simulink model "Simulation_6DOFTesting02"  (R2024a)
settings: Solver=ode4  StartTime=initial_time  StopTime=final_time  FixedStep=timestep  RelTol=1e-3
values from neighbouring files (symbols this model uses):
  aEarth = 0    [CodeTesting_6DOF.m]    (also in Constants_6DOF.m = 6378137; Constants_6DOFTesting.m = 6378137)
  alphaArray = [-30, -25, -20, -15, -10, -5, 0, 5, 10, 15, 20, 25, 30]    [CodeTesting_6DOF.m]    (also in Constants_6DOF.m; Constants_6DOFTesting.m)
  altitudeArray = [0, 1000, 2000, 3000, 4000, 5000, 6000, 7000, 8000, 9000, 10000, 15000, 20000,      25000, 30000, 35000, 40000, 45000, 50000, 55000, 60000]    [CodeTesting_6DOF.m]    (also in Constants_6DOF.m; Constants_6DOFTesting.m)
  bEarth = 0    [CodeTesting_6DOF.m]    (also in Constants_6DOF.m = 6356752.3; Constants_6DOFTesting.m = 6356752.3)
  cD_3DArray = zeros(numAoAs, numMachs, numAltitudes)    [CodeTesting_6DOF.m]    (also in Constants_6DOF.m; Constants_6DOFTesting.m)
  cL_3DArray = zeros(numAoAs, numMachs, numAltitudes)    [CodeTesting_6DOF.m]    (also in Constants_6DOF.m; Constants_6DOFTesting.m)
  densityList = rhoList    [CodeTesting_6DOF.m]    (also in Constants_6DOF.m = usAtmosphere.x_; Constants_6DOFTesting.m = usAtmosphere.x_)
  height0 = 0    [Constants_6DOF.m]    (also in Constants_6DOFTesting.m = 5000)
  heightsList = usAtmosphere.Z    [CodeTesting_6DOF.m]    (also in Constants_6DOF.m; Constants_6DOFTesting.m)
  inertialPitch0 = deg2rad(inertialPitch0)    [Constants_6DOFTesting.m]
  inertialRoll0 = deg2rad(inertialRoll0)    [Constants_6DOFTesting.m]
  inertialYaw0 = deg2rad(inertialYaw0)    [Constants_6DOFTesting.m]
  initQuatVector0 = [e0; e1; e2; e3]    [Constants_6DOFTesting.m]
  Ixx = 10    [CodeTesting_6DOF.m]    (also in Constants_6DOF.m; Constants_6DOFTesting.m = 4.88094462)
  Ixz = 10    [CodeTesting_6DOF.m]    (also in Constants_6DOF.m = 1; Constants_6DOFTesting.m = 4.88094462)
  Iyy = 10    [CodeTesting_6DOF.m]    (also in Constants_6DOF.m; Constants_6DOFTesting.m = 4.88094462)
  Izz = 10    [CodeTesting_6DOF.m]    (also in Constants_6DOF.m; Constants_6DOFTesting.m = 4.88094462)
  latitude0 = pi/4    (= 0.785398163397)    [CodeTesting_6DOF.m]    (also in Constants_6DOF.m = deg2rad(latitude0); Constants_6DOFTesting.m = deg2rad(latitude0))
  longitude0 = pi/4    (= 0.785398163397)    [CodeTesting_6DOF.m]    (also in Constants_6DOF.m = deg2rad(longitude0); Constants_6DOFTesting.m = deg2rad(longitude0))
  m0 = 10    [CodeTesting_6DOF.m]    (also in Constants_6DOF.m = 50; Constants_6DOFTesting.m = 14.5939029)
  machArray = [0.5, 1.0, 1.5, 2.0, 2.5, 3.0, 3.5, 4.0, 4.5, 5.0, 5.5, 6.0, 6.5, 7.0, 7.5, 8.0,      8.5, 9.0, 9.5, 10.0]    [CodeTesting_6DOF.m]    (also in Constants_6DOF.m; Constants_6DOFTesting.m)
  omegaEarth = omega_earth    (= 7.2921159e-05)    [CodeTesting_6DOF.m]    (also in Constants_6DOF.m; Constants_6DOFTesting.m)
  p0Body = deg2rad(p0Body)    [Constants_6DOFTesting.m]
  pitchCharacteristicLength = 0.0    (= 0)    [Constants_6DOFTesting.m]
  q0Body = deg2rad(q0Body)    [Constants_6DOFTesting.m]
  r0Body = deg2rad(r0Body)    [Constants_6DOFTesting.m]
  rEarth = r_earth    (= 6371008.8)    [CodeTesting_6DOF.m]    (also in Constants_6DOF.m; Constants_6DOFTesting.m)
  rollCharacteristicLength = 0.0    (= 0)    [Constants_6DOFTesting.m]
  temperatureList = usAtmosphere.T    [CodeTesting_6DOF.m]    (also in Constants_6DOF.m; Constants_6DOFTesting.m)
  u0Body = 304.8    [Constants_6DOFTesting.m]
  v0Body = 0    [Constants_6DOFTesting.m]
  w0Body = -1 * w0Body    (= 0)    [Constants_6DOFTesting.m]
  wingArea = 0    [CodeTesting_6DOF.m]    (also in Constants_6DOF.m = 50; Constants_6DOFTesting.m = 0.09290304)
  yawCharacteristicLength = 0.0    (= 0)    [Constants_6DOFTesting.m]
undefined symbols (not defined in the file or in its folder): inertialX0, inertialY0, inertialZ0
libraries: simulink_extras x24
(part 2 of 2)

== matlab function Simulation_6DOFTesting02/Equations of Motion/Subsystem1/MATLAB Function1 ==
  data: angularRatesBody input; y output; quatRotBTN input
function y= fcn(angularRatesBody, quatRotBTN)

rotationMatrixIB = quatRotBTN;

angularRatesInertial =  angularRatesBody;

y = angularRatesInertial;

== matlab function Simulation_6DOFTesting02/Atmospheric Conditions/Mach ==
  data: v input; y output; r input; hList input; tempList input
function y = fcn(v, r, hList, tempList)

gamma = 1.4;
rGas = 287.05;

r = r / 10^3;

if r >= 0
    temp = interp1(hList, tempList, r);
    a = sqrt(gamma * rGas * temp);
    y = v/a;
else
    temp = 0;
    y = 0;
end

== matlab function Simulation_6DOFTesting02/Forces, Moments & their Coefficients/rollMoment ==
  data: rho input; y output; v input; A input; length input; rollCoeff input
function y = fcn(rho, v, A, length, rollCoeff)

rollMoment = 0.5 * rho * v^2 * A * rollCoeff * length;

y = rollMoment;

== matlab function Simulation_6DOFTesting02/Forces, Moments & their Coefficients/pitchMoment ==
  data: rho input; y output; v input; A input; length input; pitchCoeff input
function y = fcn(rho, v, A, length, pitchCoeff)

pitchMoment = 0.5 * rho * v^2 * A * length * pitchCoeff;

y = pitchMoment;

== matlab function Simulation_6DOFTesting02/Equations of Motion/Subsystem2/MATLAB Function ==
  data: quatVector input; y output
function y = fcn(quatVector)

lambda = 1000;

quatVectorNormalized = quatVector - lambda * (1 - norm(quatVector)^2 )^2;

normQuatVecCheck = norm(quatVectorNormalized);

y = quatVectorNormalized;

== matlab function Simulation_6DOFTesting02/Forces, Moments & their Coefficients/yawMoment ==
  data: rho input; y output; v input; A input; length input; yawCoeff input
function y = fcn(rho, v, A, length, yawCoeff)

yawMoment = 0.5 * rho * v^2 * A * length * yawCoeff;

y = yawMoment;

== matlab function Simulation_6DOFTesting02/Equations of Motion/Subsystem/Subsystem4/uDot_Body ==
  data: Fx input; y output; m input; r input; v input; q input; w input
function y = fcn(Fx, m, r, v, q, w)

uDot_Wind = (Fx/m) + r * v - q * w;

y = uDot_Wind;

== matlab function Simulation_6DOFTesting02/Equations of Motion/Subsystem/Subsystem3/vDot_Body ==
  data: Fy input; y output; m input; p input; w input; r input; u input
function y = fcn(Fy, m, p, w, r,  u)

vDot_Wind = (Fy / m) + p * w - r * u;

y = vDot_Wind;

== matlab function Simulation_6DOFTesting02/Equations of Motion/Subsystem/Subsystem2/wDot_Body ==
  data: Fz input; y output; m input; q input; u input; p input; v input
function y = fcn(Fz, m, q, u, p, v)

vDot_Wind = (Fz / m) + q * u - p * v;

y = vDot_Wind;

== matlab function Simulation_6DOFTesting02/Equations of Motion/Subsystem/Subsystem/pDot_Body ==
  data: rollMoment input; y output; Ixx input; Ixz input; rDot_Body input; Izz input; Iyy input; q input; r input; p input
function y = fcn(rollMoment, Ixx, Ixz, rDot_Body, Izz, Iyy, q, r, p)

pDot_Wind = (1/Ixx) * (Ixz * rDot_Body - (Izz - Iyy) * q * r + Ixz * p * q - rollMoment);

y = pDot_Wind;

== matlab function Simulation_6DOFTesting02/Forces, Moments & their Coefficients/Subsystem1/MATLAB Function ==
  data: m input; y output; g input; quatRotBTN input
function y = fcn(m, g, quatRotBTN)

inertialGravity = [0; 0; m * g];

rotationMatrixBI = quatRotBTN;

rotationBI = inv(rotationMatrixBI);

bodyGravity = rotationBI * inertialGravity;

y = bodyGravity;

== matlab function Simulation_6DOFTesting02/Equations of Motion/Subsystem/qBody/qDot_Body ==
  data: pitchMoment input; Iyy input; Izz input; y output; Ixx input; p input; r input; Ixz input
function y = fcn(pitchMoment, Iyy, Izz, Ixx, p, r, Ixz)

qDot_Wind = (1/Iyy) * ( -pitchMoment - (Ixx - Izz) * p * r - Ixz * (p^2 - r^2));

y = qDot_Wind;

== matlab function Simulation_6DOFTesting02/Equations of Motion/Subsystem/rBody/rDot_Body ==
  data: yawMoment input; Izz input; Ixz input; pDot_Body input; y output; Ixx input; Iyy input; p input; q input; r input
function y = fcn(yawMoment, Izz, Ixz, pDot_Body, Ixx, Iyy, p, q, r)

rDot_Wind = (1/Izz) * (Ixz * pDot_Body - (Iyy - Ixx) * p * q - Ixz * q * r - yawMoment);

y = rDot_Wind;

== matlab function Simulation_6DOFTesting02/Atmospheric Conditions/g ==
  data: y output; r input
function y = fcn(r)

mu_earth = 3.986004418 * 10^14;
rE = 6378140;

y = mu_earth / (rE + r)^2;

== matlab function Simulation_6DOFTesting02/Atmospheric Conditions/rho ==
  data: rhoList input; hList input; r input; y output
function y = fcn(rhoList, hList, r)

r = r / 10^3;

if r >= 0
    density = interp1(hList, rhoList, r);
else
    density = 0;
end


y = density;

== matlab function Simulation_6DOFTesting02/Coordinate Transformations/Subsystem/velocity ==
  data: u input; y output; v input; w input
function y = fcn(u, v, w)

velocity = sqrt(u^2 + v^2 + w^2);

y = velocity;

== matlab function Simulation_6DOFTesting02/Constants & Aircraft Parameters/mass ==
  data: t input; y output; thrustBurnRate input; m0 input
function y = fcn(t, thrustBurnRate, m0)

mass = m0 - thrustBurnRate * t;

y = mass;

== matlab function Simulation_6DOFTesting02/Forces, Moments & their Coefficients/Subsystem/AoA1 ==
  data: u input; y output; v input; w input
function y = fcn(u, v, w)

%AoA = -1 * asin(w / sqrt(u^2 + v^2 + w^2) );
AoA = atan(-w / u);

y = AoA;

== matlab function Simulation_6DOFTesting02/Control Surfaces/bankAngle ==
  data: t input; y output
function y = fcn(t)

bankAngle = 0;

y = bankAngle;

== matlab function Simulation_6DOFTesting02/Control Surfaces/flightPathAngle ==
  data: t input; y output
function y = fcn(t)

flightPathAngle = 0;

y = flightPathAngle;

== matlab function Simulation_6DOFTesting02/Control Surfaces/pitchSurfaceDeflection ==
  data: t input; y output
function y = fcn(t)

pitchSurfaceDeflection = 0.0;

if t > 5 && t < 15
    pitchSurfaceDeflection = 0.001;
end

if t > 20 && t < 25
    pitchSurfaceDeflection = -0.001;
end


y = pitchSurfaceDeflection;

== matlab function Simulation_6DOFTesting02/Equations of Motion/Subsystem2/quatVectorDot ==
  data: quatVector input; y output; p input; q input; r input
function y = fcn(quatVector, p, q, r)



row1 = 1/2 * [0 -p -q -r];
row2 = 1/2 * [p 0 r -q];
row3 = 1/2 * [q -r 0 p];
row4 = 1/2 * [r q -p 0];


updateMatrix = [row1; row2; row3; row4];

quatDotVector = (updateMatrix * quatVector); 
%Normalize post integrtation - lambda * (1 - norm(quatVector)^2 )^2;

y = quatDotVector;

== matlab function Simulation_6DOFTesting02/Forces, Moments & their Coefficients/rollCoeff ==
  data: rollSurfaceDeflection input; y output
function y = fcn(rollSurfaceDeflection)

staticRollCoeff = rollSurfaceDeflection;
dynamicRollCoeff = 0.0;

rollCoeff = staticRollCoeff + dynamicRollCoeff;

y = rollCoeff;

== matlab function Simulation_6DOFTesting02/Forces, Moments & their Coefficients/pitchCoeff ==
  data: pitchSurfaceDeflection input; y output
function y = fcn(pitchSurfaceDeflection)

staticPitchCoeff = pitchSurfaceDeflection;
dynamicPitchCoeff = 0.0;

pitchCoeff = staticPitchCoeff + dynamicPitchCoeff;

y = pitchCoeff;

== matlab function Simulation_6DOFTesting02/Forces, Moments & their Coefficients/yawCoeff ==
  data: yawSurfaceDeflection input; y output
function y = fcn(yawSurfaceDeflection)

staticYawCoeff = yawSurfaceDeflection;
dynamicYawCoeff = 0.0;

yawCoeff = staticYawCoeff + dynamicYawCoeff;

y = yawCoeff;

== matlab function Simulation_6DOFTesting02/Constants & Aircraft Parameters/thrustBurnRate ==
  data: t input; y output
function y = fcn(t)

thrustBurnRate = 0;

y = thrustBurnRate;

== matlab function Simulation_6DOFTesting02/Forces, Moments & their Coefficients/Fx ==
  data: thrustX input; y output; gravityX input; dragX input
function y = fcn(thrustX, gravityX, dragX)

xForce = thrustX - gravityX - dragX;

y = xForce;

== matlab function Simulation_6DOFTesting02/Forces, Moments & their Coefficients/Fy ==
  data: thrustY input; y output; gravityY input
function y = fcn(thrustY, gravityY)

yForce = thrustY - gravityY;

y = yForce;

== matlab function Simulation_6DOFTesting02/Forces, Moments & their Coefficients/Fz ==
  data: thrustZ input; y output; gravityZ input; liftZ input
function y = fcn(thrustZ, gravityZ, liftZ)

zForce = thrustZ + gravityZ - liftZ;

y = zForce;

== matlab function Simulation_6DOFTesting02/Forces, Moments & their Coefficients/MATLAB Function ==
  data: thrustX input; y output; thrustY input; thrustZ input
function y = fcn(thrustX, thrustY, thrustZ)

thrustMagnitude = sqrt(thrustX^2 + thrustY^2 + thrustZ^2);

y = thrustMagnitude;

== matlab function Simulation_6DOFTesting02/Forces, Moments & their Coefficients/MATLAB Function1 ==
  data: forceVector input; y output; quatRotWTB input
function y = fcn(forceVector, quatRotWTB)

rotationMatrix = quatRotWTB;

rotatedForceVector = rotationMatrix * forceVector;

y = rotatedForceVector;

== matlab function Simulation_6DOFTesting02/Forces, Moments & their Coefficients/Subsystem1/MATLAB Function2 ==
  data: bodyGravity input; quatRotWTB input; y output
function y = fcn(bodyGravity, quatRotWTB)

rotationWB = inv(quatRotWTB);

windGravity = rotationWB * bodyGravity;

y = windGravity;

== matlab function Simulation_6DOFTesting02/Control Surfaces/rollSurfaceDeflection ==
  data: t input; y output
function y = fcn(t)

rollSurfaceDeflection = 0.0;

y = rollSurfaceDeflection;

== matlab function Simulation_6DOFTesting02/Control Surfaces/thrust_AoA ==
  data: t input; y output
function y = fcn(t)

thrustAoA = 0;

y = thrustAoA;

== matlab function Simulation_6DOFTesting02/Forces, Moments & their Coefficients/Subsystem/sideslipAngle1 ==
  data: u input; y output; v input; w input
function y = fcn(u, v, w)

sideslipAngle = asin(v / sqrt(u^2 + v^2 + w^2) );
%sideslipAngle = atan(u / v);

y = sideslipAngle;

== matlab function Simulation_6DOFTesting02/Equations of Motion/Subsystem2/quat2phi ==
  data: quatVector input; y output
function y = fcn(quatVector)

e0 = quatVector(1);
e1 = quatVector(2);
e2 = quatVector(3);
e3 = quatVector(4);

input1 = e0^2 + e1^2 - e1^2 - e2^2;
input2 = 2 * (e0 * e1 + e2 * e3);

phi = atan2(input2, input1);

y = phi;

== matlab function Simulation_6DOFTesting02/Equations of Motion/Subsystem2/MATLAB Function3 ==
  data: omegaEarth input; y output; latitude input; longitude input; positionNED input
function y = fcn(omegaEarth, latitude, longitude, positionNED)

omegaEarth = [0; 0; omegaEarth];
omegaEarth = [0; 0; 0];

lat = latitude;
long = longitude;

row1 = [-cos(long) * sin(lat) -sin(long) -cos(lat) * cos(long)];
row2 = [-sin(lat) * sin(long) cos(long) -cos(lat) * sin(long)];
row3 = [cos(lat) 0 -sin(lat)];

rotationMatrix = inv([row1; row2; row3]);
velocityNEDFrame = rotationMatrix * omegaEarth;
positionNED = positionNED;

velNEDX = velocityNEDFrame(1);
velNEDY = velocityNEDFrame(2);
velNEDZ = velocityNEDFrame(3);

posNEDX = positionNED(1);
posNEDY = positionNED(2);
posNEDZ = positionNED(3);

velRotEarthX = velNEDY * posNEDZ - velNEDZ * posNEDY;
velRotEarthY = velNEDZ * posNEDX - velNEDX * posNEDZ;
velRotEarthZ = velNEDX * posNEDY - velNEDY * posNEDX;

velocityRotatingEarth = [velRotEarthX; velRotEarthY; velRotEarthZ];

y = velocityRotatingEarth;

== matlab function Simulation_6DOFTesting02/Equations of Motion/Subsystem2/MATLAB Function4 ==
  data: velocityRotatingEarth input; y output
function y = fcn(velocityRotatingEarth)

magnitudeRotatingEarth = norm(velocityRotatingEarth);

y = magnitudeRotatingEarth;

== matlab function Simulation_6DOFTesting02/Control Surfaces/thrust_Sideslip ==
  data: t input; y output
function y = fcn(t)

thrustSideslip = 0;

y = thrustSideslip;

== matlab function Simulation_6DOFTesting02/Coordinate Transformations/Polar ECEF - lat, long, height/MATLAB Function ==
  data: a input; y output; b input; xECEF input; yECEF input; latitude input; height0 input
function y = fcn(a, b, xECEF, yECEF, latitude, height0)

e = sqrt(1 - b^2/a^2);
p = sqrt(xECEF^2 + yECEF^2);

N = a / sqrt(1 - e^2 * sin(latitude)^2);
alt = -1 * (p / cos(latitude) - (N + height0));


y = alt;

== matlab function Simulation_6DOFTesting02/Coordinate Transformations/Cartesian ECEF - x, y, z/MATLAB Function4 ==
  data: positionECEF input; y output
function y = fcn(positionECEF)

rEarth = 6371.0088 * 10^3;

height = norm(positionECEF) - rEarth;

y = height;

== matlab function Simulation_6DOFTesting02/Control Surfaces/yawSurfaceDeflection ==
  data: t input; y output
function y = fcn(t)

yawSurfaceDeflection = 0;

y = yawSurfaceDeflection;

== matlab function Simulation_6DOFTesting02/Coordinate Transformations/Cartesian ECEF - x, y, z/MATLAB Function ==
  data: u input; y output
function y = fcn(u)

y = norm(u);

== matlab function Simulation_6DOFTesting02/Coordinate Transformations/Polar ECEF - lat, long, height/MATLAB Function4 ==
  data: u input; y output
function y = fcn(u)

y = norm(u);

== matlab function Simulation_6DOFTesting02/Coordinate Transformations/Polar ECEF - lat, long, height/MATLAB Function5 ==
  data: latitude input; longitude input; positionNED input; y output; latitude0 input; longitude0 input; height0 input; a input; b input; t input
function y = fcn( latitude, longitude, positionNED, latitude0, longitude0, height0, a, b, t)

rEarth = 6371.0088 * 10^3; 

long = longitude;
lat = latitude;

row1 = [-cos(long) * sin(lat) -sin(long) -cos(lat) * cos(long)];
row2 = [-sin(lat) * sin(long) cos(long) -cos(lat) * sin(long)];
row3 = [cos(lat) 0 -sin(lat)];

rotationMatrix = [row1; row2; row3];

e = sqrt(1 - b^2/a^2);
N = a * (1 - e^2 * sin(latitude0)^2)^(-1/2);

initialECEFX = (height0 + N) * cos(latitude0) * cos(longitude0);
initialECEFY = (height0 + N) * cos(latitude0) * sin(longitude0);
initialECEFZ = (height0 + N * (1 - e^2)) * sin(latitude0);

initialECEFPosition = [initialECEFX; initialECEFY; initialECEFZ];


positionECEF = rotationMatrix * positionNED + initialECEFPosition;

y = positionECEF;

== matlab function Simulation_6DOFTesting02/Equations of Motion/Subsystem2/quatRotMatrix ==
  data: quatVector input; y output
function y = fcn(quatVector)

e0 = quatVector(1);
e1 = quatVector(2);
e2 = quatVector(3);
e3 = quatVector(4);

a = e0;
b = e1;
c = e2;
d = e3;

aa = e0 * e0;
bb = e1 * e1;
cc = e2 * e2;
dd = e3 * e3;

s = 1 / ( aa + bb + cc + dd );
two_s = 2 * s;

row1 = [s * ( aa + bb - cc - dd ), two_s * ( b * c - a * d ), two_s * ( b * d + a * c )];
row2 = [two_s * ( b * c + a * d ), s * ( aa - bb + cc - dd ), two_s * ( c * d - a * b )];
row3 = [two_s * ( b * d - a * c ), two_s * ( c * d + a * b ), s * ( aa - bb - cc + dd )];

rotationMatrixQuat = inv([row1; row2; row3]);

y = rotationMatrixQuat;

== matlab function Simulation_6DOFTesting02/Coordinate Transformations/Polar ECEF - lat, long, height/MATLAB Function6 ==
  data: t input; y output; latitude0 input; xECEF input; yECEF input; zECEF input; a input; b input
function y = fcn(t, latitude0, xECEF, yECEF, zECEF, a, b)

e = sqrt(1 - b^2/a^2);
e2 = sqrt(a^2/b^2 - 1);
p = sqrt(xECEF^2 + yECEF^2);

theta = atan2(zECEF * a, p * b);
lat = atan2(zECEF + e2^2 * b * sin(theta)^3, p - e^2 * a * cos(theta)^3);

if t == 0
    latitude = latitude0;
else
    latitude = lat;
end

y = latitude;

== matlab function Simulation_6DOFTesting02/Coordinate Transformations/Polar ECEF - lat, long, height/MATLAB Function7 ==
  data: t input; y output; longitude0 input; xECEF input; yECEF input
function y = fcn(t, longitude0, xECEF, yECEF)

long = atan2(yECEF, xECEF);

if t == 0
    long = longitude0;
else
    long = atan2(yECEF, xECEF);
end

longitude = long;

y = longitude;

== matlab function Simulation_6DOFTesting02/Forces, Moments & their Coefficients/Subsystem/MATLAB Function ==
  data: vNED input; y output; quatRotBTN input
function y = fcn(vNED, quatRotBTN)

vBody = inv(quatRotBTN) * vNED;

y = vBody;

== matlab function Simulation_6DOFTesting02/Equations of Motion/Subsystem2/quat2psi ==
  data: quatVector input; y output
function y = fcn(quatVector)

e0 = quatVector(1);
e1 = quatVector(2);
e2 = quatVector(3);
e3 = quatVector(4);

input1 = e0^2 + e1^2 - e2^2 - e3^3;
input2 = 2 * (e0 * e3 + e1 * e2);

psi = atan2(input2, input1);

y = psi;

== matlab function Simulation_6DOFTesting02/Equations of Motion/Subsystem2/quat2theta ==
  data: quatVector input; y output
function y = fcn(quatVector)

e0 = quatVector(1);
e1 = quatVector(2);
e2 = quatVector(3);
e3 = quatVector(4);

input = 2 * (e0 * e2 - e1 * e3);

theta = asin(input);

y = theta;

== matlab function Simulation_6DOFTesting02/Forces, Moments & their Coefficients/DragX ==
  data: rho input; y output; v input; cd input; A input
function y = fcn(rho, v, cd, A)

cd = 0.1;
Drag = 0.5 * rho * v^2 * A * cd;

y = Drag;
y = 0;

== matlab function Simulation_6DOFTesting02/Forces, Moments & their Coefficients/LiftZ ==
  data: rho input; y output; cl input; A input; v input
function y = fcn(rho, cl, A, v)

Lift =  0.5 * rho * v^2 * A * cl;
Lift = 0;

y = Lift;

== matlab function Simulation_6DOFTesting02/Forces, Moments & their Coefficients/thrustX ==
  data: t input; y output; thrustAoA input; thrustSideslip input; quatRotWTB input
function y = fcn(t, thrustAoA, thrustSideslip, quatRotWTB)

thrust = 0;

thrust = thrust * cos(thrustAoA) * cos(thrustSideslip);

thrustVector = [thrust; 0; 0];

thrustWind = inv(quatRotWTB) * thrustVector;

thrustWindX = thrustWind(1);

y = thrustWindX;
